simulink library "Environment_cl"  (R2020a)
settings: Solver=VariableStepAuto  StartTime=0.0  StopTime=10.0  RelTol=1e-3
undefined symbols (not defined in the file): Env
libraries: AirDensity_ul x1, StopSim_ul x1, LinWindSpeed_ul x1
settings Model: Creator=jbore  LastModifiedBy=bunce
settings SFSimCC: CustomCodeUndefinedFunction=UseInterfaceOnly

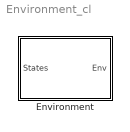
== system Environment_cl ==
  Environment : Subsystem
      mask Display:
      | patch([0 1 1 0], [0 0 1 1],[1 .85 1])
      | 
      | port_label('input',1,'States','texmode','on')
      | 
      | port_label('output',1,'Env','texmode','on')

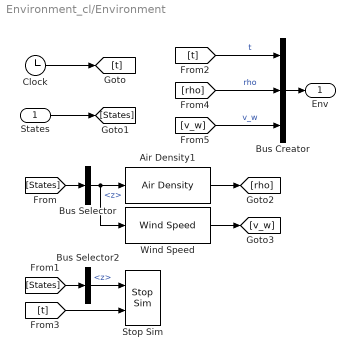
== system Environment_cl/Environment ==
  States : Inport
  Air Density1 : AirDensity_ul/Air Density  rho=Env.rho  g=Env.g  M=Env.M  R=Env.R  T_0=Env.T_0
  Bus Creator : BusCreator  Inputs=3
  Bus Selector : BusSelector  OutputSignals=z
  Bus Selector2 : BusSelector  OutputSignals=z
  Clock : Clock
  Stop Sim : StopSim_ul/Stop Sim  z_0=Env.z_0  t_b=Mot.t_b
  Wind Speed : LinWindSpeed_ul/Wind Speed  v0=Env.v_w1  v1=Env.v_w2  h0=Env.z_0  h1=Env.z_w
  Env : Outport  VectorParamsAs1DForOutWhenUnconnected=off
  wires:
  Bus Creator/1 -> Env/1
  Clock/1 -> [t]
  [t] -> Bus Creator/1  "t"
  States/1 -> [States]
  [States] -> Bus Selector/1
  Bus Selector/1 -> Wind Speed/1, Air Density1/1  "<z>"
  Air Density1/1 -> [rho]
  [rho] -> Bus Creator/2  "rho"
  [States] -> Bus Selector2/1
  Bus Selector2/1 -> Stop Sim/1  "<z>"
  [t] -> Stop Sim/2
  Wind Speed/1 -> [v_w]
  [v_w] -> Bus Creator/3  "v_w"
